simulink model "Clutch_Model"  (R2020b)
settings: Solver=VariableStepAuto  StartTime=0.0  StopTime=10.0  RelTol=1e-3
undefined symbols (not defined in the file): be, bv, Ie, Iv, muk, mus, R
settings Model: Creator=Rasika Shejul  LastModifiedBy=Rasika Shejul

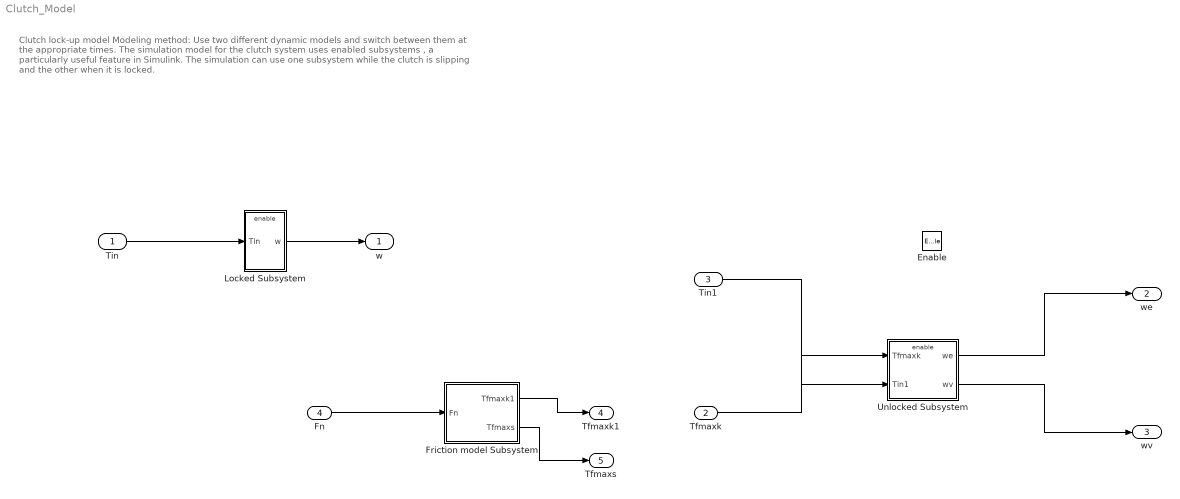
== system Clutch_Model ==
  note: Clutch lock-up model
      | Modeling method: Use two different dynamic models and switch between them at the appropriate times. The simulation model for the clutch system uses enabled subsystems , a particularly useful feature in Simulink. The simulation can use one subsystem while the clutch is slipping and the other when it is locked.
  Tin : Inport
  Tfmaxk : Inport  Port=2
  Tin1 : Inport  Port=3
  Fn : Inport  Port=4
  Enable : EnablePort  StatesWhenEnabling=reset
  Friction model Subsystem : Subsystem
  Locked Subsystem : Subsystem
  Unlocked Subsystem : Subsystem
  w : Outport  InitialOutput=0  VectorParamsAs1DForOutWhenUnconnected=off
  we : Outport  Port=2  InitialOutput=0  VectorParamsAs1DForOutWhenUnconnected=off
  wv : Outport  Port=3  InitialOutput=0  VectorParamsAs1DForOutWhenUnconnected=off
  Tfmaxk1 : Outport  Port=4  InitialOutput=0  VectorParamsAs1DForOutWhenUnconnected=off
  Tfmaxs : Outport  Port=5  InitialOutput=0  VectorParamsAs1DForOutWhenUnconnected=off
  wires:
  Tin/1 -> Locked Subsystem/1(Tin)
  Locked Subsystem/1(w) -> w/1
  Tfmaxk/1 -> Unlocked Subsystem/1(Tfmaxk)
  Tin1/1 -> Unlocked Subsystem/2(Tin1)
  Unlocked Subsystem/1(we) -> we/1
  Unlocked Subsystem/2(wv) -> wv/1
  Fn/1 -> Friction model Subsystem/1(Fn)
  Friction model Subsystem/1(Tfmaxk1) -> Tfmaxk1/1
  Friction model Subsystem/2(Tfmaxs) -> Tfmaxs/1

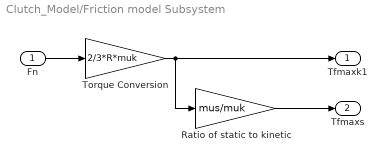
== system Clutch_Model/Friction model Subsystem ==
  Fn : Inport
  Ratio of static to kinetic : Gain  Gain=mus/muk  SaturateOnIntegerOverflow=on  OutDataTypeStr=Inherit: Same as input  ParamDataTypeStr=Inherit: Same as input
  Torque Conversion : Gain  Gain=2/3*R*muk  SaturateOnIntegerOverflow=on  OutDataTypeStr=Inherit: Same as input  ParamDataTypeStr=Inherit: Same as input
  Tfmaxk1 : Outport  InitialOutput=0  VectorParamsAs1DForOutWhenUnconnected=off
  Tfmaxs : Outport  Port=2  InitialOutput=0  VectorParamsAs1DForOutWhenUnconnected=off
  wires:
  Torque Conversion/1 -> Tfmaxk1/1, Ratio of static to kinetic/1
  Fn/1 -> Torque Conversion/1
  Ratio of static to kinetic/1 -> Tfmaxs/1

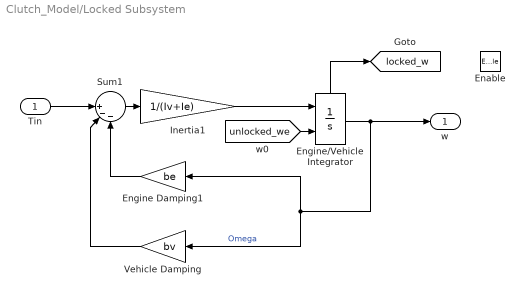
== system Clutch_Model/Locked Subsystem ==
  Tin : Inport
  Enable : EnablePort
  Engine Damping1 : Gain  Gain=be  SaturateOnIntegerOverflow=on  OutDataTypeStr=Inherit: Same as input  ParamDataTypeStr=Inherit: Same as input
  Engine/Vehicle Integrator : Integrator  InitialConditionSource=external  ShowStatePort=on
  Inertia1 : Gain  Gain=1/(Iv+Ie)  SaturateOnIntegerOverflow=on  OutDataTypeStr=Inherit: Same as input  ParamDataTypeStr=Inherit: Same as input
  Sum1 : Sum  Inputs=||+--  InputSameDT=on  SaturateOnIntegerOverflow=on  OutDataTypeStr=Inherit: Same as first input
  Vehicle Damping : Gain  Gain=bv  SaturateOnIntegerOverflow=on  OutDataTypeStr=Inherit: Same as input  ParamDataTypeStr=Inherit: Same as input
  w : Outport  InitialOutput=0  VectorParamsAs1DForOutWhenUnconnected=off
  tag scope: locked_w=global
  wires:
  Engine Damping1/1 -> Sum1/3
  Engine/Vehicle Integrator/1 -> w/1, Engine Damping1/1, Vehicle Damping/1  "Omega"
  [unlocked_we] -> Engine/Vehicle Integrator/2
  Sum1/1 -> Inertia1/1
  Tin/1 -> Sum1/1
  Vehicle Damping/1 -> Sum1/2
  Engine/Vehicle Integrator/State -> [locked_w]
  Inertia1/1 -> Engine/Vehicle Integrator/1

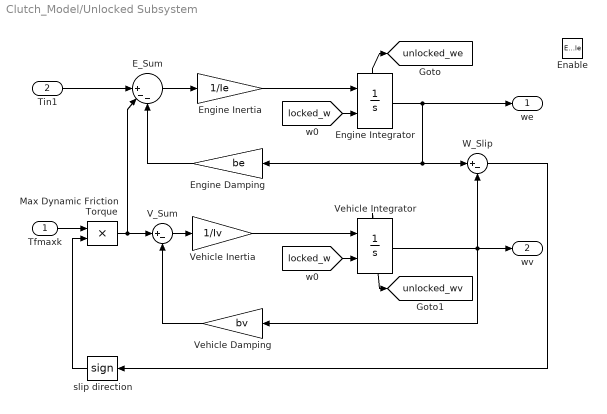
== system Clutch_Model/Unlocked Subsystem ==
  Tfmaxk : Inport
  Tin1 : Inport  Port=2
  Enable : EnablePort
  E_Sum : Sum  Inputs=||+--  InputSameDT=on  SaturateOnIntegerOverflow=on  OutDataTypeStr=Inherit: Same as first input
  Engine Damping : Gain  Gain=be  SaturateOnIntegerOverflow=on  OutDataTypeStr=Inherit: Same as input  ParamDataTypeStr=Inherit: Same as input
  Engine Inertia : Gain  Gain=1/Ie  SaturateOnIntegerOverflow=on  OutDataTypeStr=Inherit: Same as input  ParamDataTypeStr=Inherit: Same as input
  Engine Integrator : Integrator  InitialConditionSource=external  ShowStatePort=on
  Max Dynamic Friction Torque : Product  InputSameDT=on  RndMeth=Zero  SaturateOnIntegerOverflow=on  OutDataTypeStr=Inherit: Same as first input
  V_Sum : Sum  Inputs=|+-  InputSameDT=on  SaturateOnIntegerOverflow=on  OutDataTypeStr=Inherit: Same as first input
  Vehicle Damping : Gain  Gain=bv  SaturateOnIntegerOverflow=on  OutDataTypeStr=Inherit: Same as input  ParamDataTypeStr=Inherit: Same as input
  Vehicle Inertia : Gain  Gain=1/Iv  SaturateOnIntegerOverflow=on  OutDataTypeStr=Inherit: Same as input  ParamDataTypeStr=Inherit: Same as input
  Vehicle Integrator : Integrator  InitialConditionSource=external  ShowStatePort=on
  W_Slip : Sum  Inputs=|+-  InputSameDT=on  SaturateOnIntegerOverflow=on  OutDataTypeStr=Inherit: Same as first input
  slip direction : Signum
  we : Outport  InitialOutput=0  VectorParamsAs1DForOutWhenUnconnected=off
  wv : Outport  Port=2  InitialOutput=0  VectorParamsAs1DForOutWhenUnconnected=off
  tag scope: unlocked_we=global, unlocked_wv=global
  wires:
  E_Sum/1 -> Engine Inertia/1
  Vehicle Integrator/1 -> wv/1, W_Slip/2, Vehicle Damping/1
  Vehicle Integrator/State -> [unlocked_wv]
  Engine Integrator/1 -> we/1, Engine Damping/1, W_Slip/1
  Vehicle Inertia/1 -> Vehicle Integrator/1
  [locked_w] -> Vehicle Integrator/2
  Tfmaxk/1 -> Max Dynamic Friction Torque/1
  W_Slip/1 -> slip direction/1
  Engine Inertia/1 -> Engine Integrator/1
  Vehicle Damping/1 -> V_Sum/2
  V_Sum/1 -> Vehicle Inertia/1
  slip direction/1 -> Max Dynamic Friction Torque/2
  [locked_w] -> Engine Integrator/2
  Max Dynamic Friction Torque/1 -> V_Sum/1, E_Sum/2
  Tin1/1 -> E_Sum/1
  Engine Integrator/State -> [unlocked_we]
  Engine Damping/1 -> E_Sum/3
